simulink subsystem "Scopes"  (R2025a)
settings: Solver=VariableStepAuto  StartTime=0.0  StopTime=10.0  RelTol=1e-3
libraries: simulink_extras x7, aerolibanim x1
settings Model: Creator=Andrew Radulovich  LastModifiedBy=thatf
settings ModelReferenceCC: EnableRefExpFcnMdlSchedulingChecks=on
settings RTWCC: GPUComputeCapability=3.5

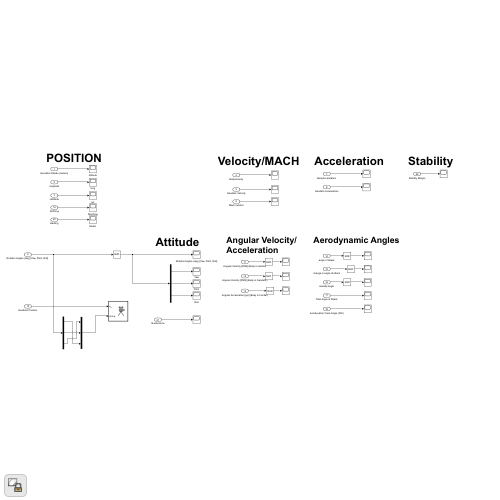
[thumbnail: Simulink's stored preview of the top-level diagram]
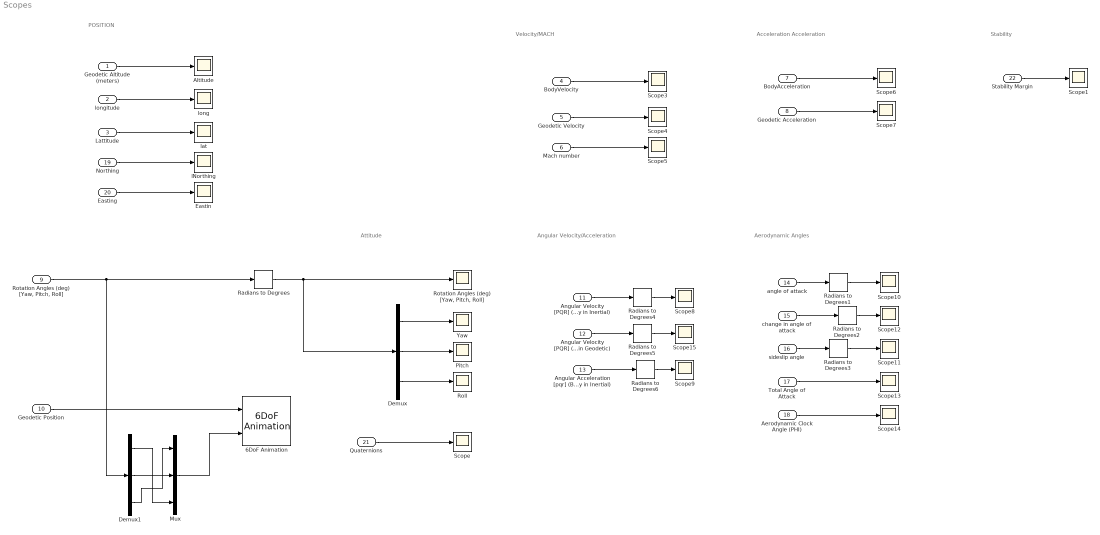
== system Scopes ==
  note: POSITION
  note: Velocity/MACH
  note: Acceleration
      | Acceleration
  note: Angular Velocity/Acceleration
  note: Attitude
  note: Aerodynamic Angles
  note: Stability
  Geodetic Altitude (meters) : Inport
  longitude : Inport  Port=2
  Lattitude : Inport  Port=3
  BodyVelocity : Inport  Port=4
  Geodetic Velocity : Inport  Port=5
  Mach number : Inport  Port=6
  BodyAcceleration : Inport  Port=7
  Geodetic Acceleration : Inport  Port=8
  "Rotation Angles (deg) [Yaw, Pitch, Roll] " : Inport  Port=9
  Geodetic Position : Inport  Port=10
  Angular Velocity [PQR] (Body in Inertial) : Inport  Port=11
  Angular Velocity [PQR] (Body in Geodetic) : Inport  Port=12
  Angular Acceleration [pqr] (Body in Inertial) : Inport  Port=13
  angle of attack : Inport  Port=14
  change in angle of attack : Inport  Port=15
  sideslip angle : Inport  Port=16
  Total Angle of Attack : Inport  Port=17
  Aerodynamic Clock Angle (PHI) : Inport  Port=18
  Northing : Inport  Port=19
  Easting : Inport  Port=20
  Quaternions : Inport  Port=21
  Stability Margin : Inport  Port=22
  6DoF Animation : aerolibanim/6DoF Animation  u1=[-10 10 -10 10 -10 10]  u2=0.1  u3=1.0  u4=[0 0 0]  u5=Fly alongside  u6=[8 -8 0]  u7=10  u8=on
  Altitude : Scope
      settings: ActiveDisplayYMinimum=-156.174960440639  ActiveDisplayYMaximum=1519.769328249482
  Demux : Demux  Outputs=3
  Demux1 : Demux  Outputs=3
  Eastin : Scope
      settings: ActiveDisplayYMinimum=-1  ActiveDisplayYMaximum=1  DataLoggingVariableName=ScopeData2
  Mux : Mux  Inputs=3
  Pitch : Scope
      settings: ActiveDisplayYMinimum=-104.2903  ActiveDisplayYMaximum=111.58781  DataLoggingVariableName=ScopeData9
  Radians to Degrees{,1..6} (7 alike) : simulink_extras/Transformations/Radians to Degrees
  Roll : Scope
      settings: ActiveDisplayYMinimum=-224.97057  ActiveDisplayYMaximum=224.99309  DataLoggingVariableName=ScopeData10
  "Rotation Angles (deg) [Yaw, Pitch, Roll]" : Scope
      settings: ActiveDisplayYMinimum=18.51521  ActiveDisplayYMaximum=55.51777  DataLoggingVariableName=ScopeData3
  Scope{,1,3..15} (15 alike) : Scope
      Scope settings: ActiveDisplayYMinimum=-0.08935  ActiveDisplayYMaximum=0.80319  DataLoggingVariableName=ScopeData4
      Scope1 settings: ActiveDisplayYMinimum=2.9035706604207663  ActiveDisplayYMaximum=3.2439600073482753  DataLoggingVariableName=ScopeData5
      Scope10 settings: ActiveDisplayYMinimum=-0.15643993270491208  ActiveDisplayYMaximum=0.22718504433416967  DataLoggingVariableName=ScopeData6
      Scope11 settings: ActiveDisplayYMinimum=-12.91032  ActiveDisplayYMaximum=34.71829  DataLoggingVariableName=ScopeData31
      Scope12 settings: ActiveDisplayYMinimum=-110.96984  ActiveDisplayYMaximum=76.07472  DataLoggingVariableName=ScopeData32
      Scope13 settings: ActiveDisplayYMinimum=-0.763315701348326  ActiveDisplayYMaximum=2.3640028093355947  DataLoggingVariableName=ScopeData33
      Scope14 settings: ActiveDisplayYMinimum=-224.73085  ActiveDisplayYMaximum=224.85317  DataLoggingVariableName=ScopeData18
      Scope15 settings: ActiveDisplayYMinimum=-70.24868  ActiveDisplayYMaximum=70.59805  DataLoggingVariableName=ScopeData19
      Scope3 settings: ActiveDisplayYMinimum=-109.7314297134609  ActiveDisplayYMaximum=263.84020546343066  DataLoggingVariableName=ScopeData20
      Scope4 settings: ActiveDisplayYMinimum=-1097.6443  ActiveDisplayYMaximum=121.9621  DataLoggingVariableName=ScopeData21
      Scope5 settings: ActiveDisplayYMinimum=0.017063795753241684  ActiveDisplayYMaximum=0.70440714159724782  DataLoggingVariableName=ScopeData22
      Scope6 settings: ActiveDisplayYMinimum=-91.080419646713608  ActiveDisplayYMaximum=294.989225068752  DataLoggingVariableName=ScopeData23
      Scope7 settings: ActiveDisplayYMinimum=-422.66587  ActiveDisplayYMaximum=117.9002  DataLoggingVariableName=ScopeData24
      Scope8 settings: ActiveDisplayYMinimum=-8.62413  ActiveDisplayYMaximum=4.10151  DataLoggingVariableName=ScopeData25
      Scope9 settings: ActiveDisplayYMinimum=-240.64026  ActiveDisplayYMaximum=31.00275  DataLoggingVariableName=ScopeData26
  Yaw : Scope
      settings: ActiveDisplayYMinimum=-224.67757  ActiveDisplayYMaximum=223.97807  DataLoggingVariableName=ScopeData27
  lNorthing : Scope
      settings: ActiveDisplayYMinimum=-1621.06612  ActiveDisplayYMaximum=180.31688  DataLoggingVariableName=ScopeData28
  lat : Scope
      settings: ActiveDisplayYMinimum=0.705529  ActiveDisplayYMaximum=0.705623  DataLoggingVariableName=ScopeData29
  long : Scope
      settings: ActiveDisplayYMinimum=-2.51693  ActiveDisplayYMaximum=-0.51693  DataLoggingVariableName=ScopeData30
  wires:
  Geodetic Altitude (meters)/1 -> Altitude/1
  longitude/1 -> long/1
  Lattitude/1 -> lat/1
  BodyVelocity/1 -> Scope3/1
  Geodetic Velocity/1 -> Scope4/1
  Mach number/1 -> Scope5/1
  BodyAcceleration/1 -> Scope6/1
  Geodetic Acceleration/1 -> Scope7/1
  Angular Velocity [PQR] (Body in Inertial)/1 -> Radians to Degrees4/1
  Angular Acceleration [pqr] (Body in Inertial)/1 -> Radians to Degrees6/1
  "Rotation Angles (deg) [Yaw, Pitch, Roll] "/1 -> Demux1/1, Radians to Degrees/1
  Demux/1 -> Yaw/1
  Demux/2 -> Pitch/1
  Demux/3 -> Roll/1
  angle of attack/1 -> Radians to Degrees1/1
  sideslip angle/1 -> Radians to Degrees3/1
  change in angle of attack/1 -> Radians to Degrees2/1
  Radians to Degrees/1 -> "Rotation Angles (deg) [Yaw, Pitch, Roll]"/1, Demux/1
  Geodetic Position/1 -> 6DoF Animation/1
  Total Angle of Attack/1 -> Scope13/1
  Aerodynamic Clock Angle (PHI)/1 -> Scope14/1
  Angular Velocity [PQR] (Body in Geodetic)/1 -> Radians to Degrees5/1
  Radians to Degrees1/1 -> Scope10/1
  Radians to Degrees2/1 -> Scope12/1
  Radians to Degrees3/1 -> Scope11/1
  Radians to Degrees4/1 -> Scope8/1
  Radians to Degrees5/1 -> Scope15/1
  Radians to Degrees6/1 -> Scope9/1
  Northing/1 -> lNorthing/1
  Easting/1 -> Eastin/1
  Quaternions/1 -> Scope/1
  Demux1/2 -> Mux/2
  Demux1/1 -> Mux/3
  Demux1/3 -> Mux/1
  Stability Margin/1 -> Scope1/1
  Mux/1 -> 6DoF Animation/2
